simulink model "Flight Control System"  (R2014a)
settings: Solver=ode45  StartTime=0.0  StopTime=100  RelTol=1e-3
libraries: simulink x1
settings Model: Creator=Asus  LastModifiedBy=Asus

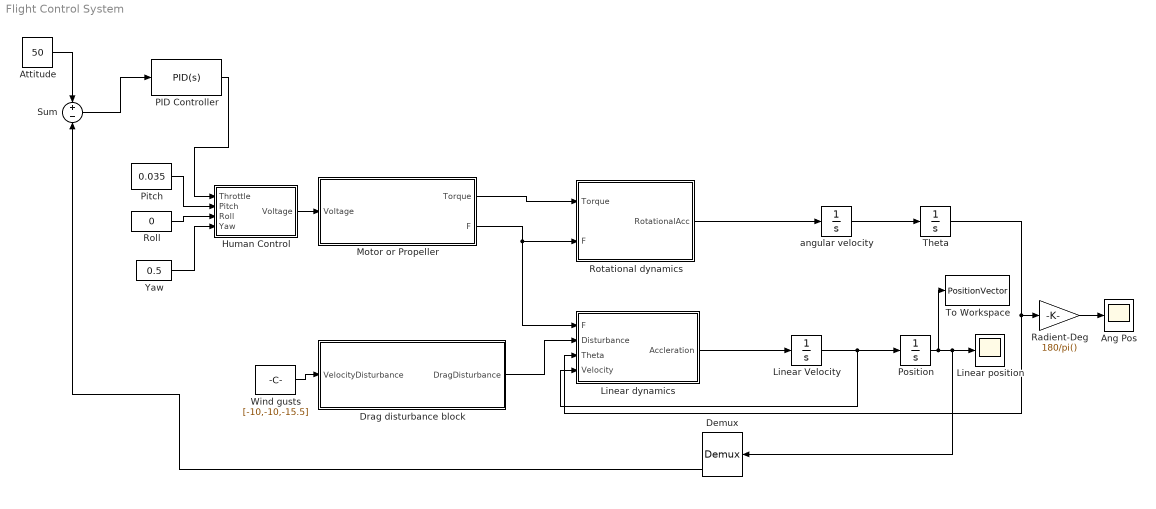
== system Flight Control System ==
  "Ang Pos " : Scope
      settings: TimeRange=10  YMin=-15000  YMax=0  SaveName=ScopeData2
  "Attitude " : Constant  Value=50
  Demux : Demux  Outputs=3
  Drag disturbance block : MATLAB Function  TreatAsAtomicUnit=on
  Human Control : MATLAB Function  TreatAsAtomicUnit=on
  "Linear position " : Scope
      settings: TickLabels=on  TimeRange=10000  YMin=0  YMax=19  SaveName=ScopeData3
  Linear Velocity : Integrator
  Linear dynamics : MATLAB Function  TreatAsAtomicUnit=on
  Motor or Propeller : MATLAB Function  TreatAsAtomicUnit=on
  PID Controller : simulink/Continuous/PID Controller  Controller=PID  TimeDomain=Continuous-time  SampleTime=1  IntegratorMethod=Forward Euler  FilterMethod=Forward Euler  Form=Parallel  P=9.031  I=0.526  D=34.39  N=100  InitialConditionSource=internal  InitialConditionForIntegrator=0  InitialConditionForFilter=0  ExternalReset=none  LimitOutput=on  UpperSaturationLimit=100  LowerSaturationLimit=0  LinearizeAsGain=on  AntiWindupMode=clamping  Kb=1  TrackingMode=off  Kt=1  PParamMin=[]  PParamMax=[]  IParamMin=[]  IParamMax=[]  DParamMin=[]  DParamMax=[]  NParamMin=[]  NParamMax=[]  KbParamMin=[]  KbParamMax=[]  KtParamMin=[]  KtParamMax=[]  POutMin=[]  POutMax=[]  IOutMin=[]  IOutMax=[]  DOutMin=[]  DOutMax=[]  NOutMin=[]  NOutMax=[]  KbOutMin=[]  KbOutMax=[]  KtOutMin=[]  KtOutMax=[]  IntegratorOutMin=[]  IntegratorOutMax=[]  FilterOutMin=[]  FilterOutMax=[]  SumOutMin=[]  SumOutMax=[]  SumI1OutMin=[]  SumI1OutMax=[]  SumI2OutMin=[]  SumI2OutMax=[]  SumI3OutMin=[]  SumI3OutMax=[]  SumDOutMin=[]  SumDOutMax=[]  SaturationOutMin=[]  SaturationOutMax=[]  IntegratorContinuousStateAttributes=''  IntegratorStateMustResolveToSignalObject=off  IntegratorRTWStateStorageClass=Auto  FilterContinuousStateAttributes=''  FilterStateMustResolveToSignalObject=off  FilterRTWStateStorageClass=Auto
  Pitch : Constant  Value=0.035
  Position : Integrator
  Radient-Deg : Gain  Gain=180/pi()
  Roll : Constant  Value=0
  "Rotational dynamics " : MATLAB Function  TreatAsAtomicUnit=on
  Sum : Sum  Inputs=+-
  "Theta " : Integrator
  To Workspace : ToWorkspace  VariableName=PositionVector  SampleTime=-1
      settings: Save2DSignal=2-D array (concatenate along first dimension)
  Wind gusts : Constant  Value=[-10,-10,-15.5]
  Yaw : Constant  Value=0.5
  angular velocity : Integrator
  wires:
  Motor or Propeller/2(F) -> "Rotational dynamics "/2(F), Linear dynamics/1(F)
  angular velocity/1 -> "Theta "/1
  "Theta "/1 -> Linear dynamics/3(Theta), Radient-Deg/1
  Linear dynamics/1(Accleration) -> Linear Velocity/1
  Linear Velocity/1 -> Linear dynamics/4(Velocity), Position/1
  Drag disturbance block/1(DragDisturbance) -> Linear dynamics/2(Disturbance)
  Wind gusts/1 -> Drag disturbance block/1(VelocityDisturbance)
  Human Control/1(Voltage) -> Motor or Propeller/1(Voltage)
  Pitch/1 -> Human Control/2(Pitch)
  Roll/1 -> Human Control/3(Roll)
  Yaw/1 -> Human Control/4(Yaw)
  Radient-Deg/1 -> "Ang Pos "/1
  Position/1 -> To Workspace/1, Demux/1, "Linear position "/1
  "Attitude "/1 -> Sum/1
  Sum/1 -> PID Controller/1
  PID Controller/1 -> Human Control/1(Throttle)
  Demux/3 -> Sum/2
  Motor or Propeller/1(Torque) -> "Rotational dynamics "/1(Torque)
  "Rotational dynamics "/1(RotationalAcc) -> angular velocity/1

== matlab function Flight Control System/Rotational dynamics  ==
  data: Torque input; F input; RotationalAcc output
function RotationalAcc=fcn(Torque,F)
Moment=[0 0 0];
RotationalAcc=[0 0 0 ];
I=[0.003,0.003,0.007];
Moment(1)=(F(3)+F(4))*0.237/2-(F(1)+F(2))*0.237/2;
Moment(2)=(F(3)+F(2))*0.237/2-(F(1)+F(4))*0.237/2;
Moment(3)=Torque(4)-Torque(1)+Torque(2)-Torque(3);
for i=1:3
    RotationalAcc(i)=Moment(i)/I(i);
end

== matlab function Flight Control System/Motor or Propeller ==
  data: Voltage input; Torque output; F output
function [Torque,F]=fcn(Voltage)
RPM=[0 0 0 0];
Torque=[0 0 0 0];
%#codegen
F=[0 0 0 0];
for i=1:4
    RPM(i)=-2.6931*Voltage(i)^3+1400*Voltage(i);
    Ct=2*10^-15*RPM(i)^3-4*10^-11*RPM(i)^2+3*10^-7*RPM(i)+0.1013;
    F(i)=Ct*1.225*(RPM(i)/60)^2*0.2^4;
    Torque(i)=4*10^-14*RPM(i)^3+8*10^-12*RPM(i)^2+3*10^-6*RPM(i);
end

== matlab function Flight Control System/Linear dynamics ==
  data: F input; Accleration output; Disturbance input; Theta input; Velocity input
function Accleration= fcn(F,Disturbance,Theta,Velocity)
M=0.743;
g=9.81;
A=[0.0197 0.0197 0.0512];
rho=1.225;
Cd=1;
Accleration=[0 0 0];
Force=[0 0 0];
Fprop=[0 0 0];
Fprop(1)=sin(Theta(2))*cos(Theta(1))*(F(1)+F(2)+F(3)+F(4));
Fprop(2)=sin(Theta(1))*cos(Theta(2))*(F(1)+F(2)+F(3)+F(4));
Fprop(3)=cos(Theta(1))*cos(Theta(2))*(F(1)+F(2)+F(3)+F(4));
ThetaXY=atan2(Fprop(1),Fprop(2)^2);
XY2D=sqrt(Fprop(1)^2+Fprop(2)^2);
if Fprop(3)>=0
    Fprop(1)=XY2D*sin(ThetaXY+Theta(3));
    Fprop(2)=XY2D*cos(ThetaXY+Theta(3));
else 
    Fprop(1)=XY2D*sin(-ThetaXY+Theta(3));
    Fprop(2)=XY2D*cos(-ThetaXY+Theta(3));
end
if Velocity(1)<0
    Force(1)=Fprop(1)-Disturbance(1)+0.5*rho*Velocity(1)^2*A(1)*Cd;
else
    Force(1)=Fprop(1)-Disturbance(1)-0.5*rho*Velocity(1)^2*A(1)*Cd;
end
if Velocity(2)<0
    Force(2)=Fprop(2)-Disturbance(2)+0.5*rho*Velocity(2)^2*A(2)*Cd;
else
    Force(2)=Fprop(2)-Disturbance(2)-0.5*rho*Velocity(2)^2*A(2)*Cd;
end
if Velocity(3)<0
    Force(3)=Fprop(3)-Disturbance(3)+0.5*rho*Velocity(3)^2*A(3)*Cd-M*g;
else
    Force(3)=Fprop(3)-Disturbance(3)-0.5*rho*Velocity(3)^2*A(3)*Cd-M*g;
end
for i=1:3
    Accleration(i)=Force(i)/M;
end

== matlab function Flight Control System/Drag disturbance block ==
  data: VelocityDisturbance input; DragDisturbance output
function DragDisturbance = fcn(VelocityDisturbance)
A=[0.0197 0.0197 0.0197*2*1.3];
DragDisturbance=[0 0 0];
roh=1.225;
Cd=1;
for i=1:3
    if VelocityDisturbance(i)<0
        DragDisturbance(i)=-0.5*roh*VelocityDisturbance(i)^2*A(i)*Cd;
    else
        DragDisturbance(i)=0.5*roh*VelocityDisturbance(i)^2*A(i)*Cd;
  
    end     
end

        
%#codegen

== matlab function Flight Control System/Human Control ==
  data: Throttle input; Voltage output; Pitch input; Roll input; Yaw input
function Voltage = fcn(Throttle,Pitch,Roll,Yaw)
Correct=0;
if(Pitch/2+Roll/2+Yaw/2)>(100-Throttle)
    Correct=((Pitch/2+Roll/2+Yaw/2)-(100-Throttle));
end
if(Pitch/2+Roll/2+Yaw/2)>(Throttle-10)
    if Correct<((Pitch/2+Roll/2+Yaw/2)-(Throttle-10))
        Correct=(Pitch/2+Roll/2+Yaw/2)-(Throttle-10);
    end
end
if Correct~=0
Pitch=Pitch-Correct/3*2;
Roll=Roll-Correct/3*2;
Yaw=Yaw-Correct/3*2;
end
Voltage=[(Throttle-Pitch/2-Roll/2-Yaw/2)*11.4/100
    (Throttle-Pitch/2+Roll/2+Yaw/2)*11.4/100
    (Throttle+Pitch/2+Roll/2-Yaw/2)*11.4/100
    (Throttle+Pitch/2-Roll/2+Yaw/2)*11.4/100];




        
    

%#codegen
